simulink model "SimulazioneCaso1_Ins_Sin"  (R2019b)
settings: Solver=VariableStepAuto  StartTime=0.0  StopTime=100  RelTol=1e-3
settings Model: Creator=sugam  LastModifiedBy=sugam

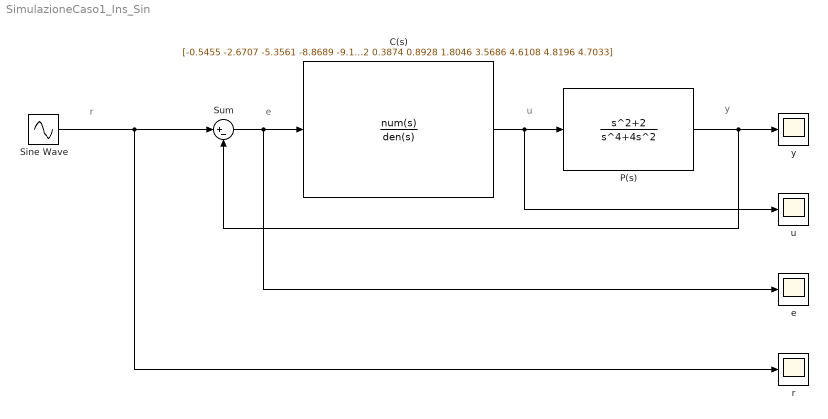
== system SimulazioneCaso1_Ins_Sin ==
  note: y
  note: u
  note: e
  note: r
  C(s) : TransferFcn  Numerator=[-0.5455 -2.6707 -5.3561 -8.8689 -9.1461 0.0529 0.0049]  Denominator=[0.0001 0.0021 0.0197 0.1092 0.3874 0.8928 1.8046 3.5686 4.6108 4.8196 4.7033]
  P(s) : TransferFcn  Numerator=[1 0 2]  Denominator=[1 0 4 0 0]
  Sine Wave : Sin  Amplitude=2  SampleTime=0
  Sum : Sum  Inputs=|+-
  e : Scope
  r : Scope
  u : Scope
  y : Scope
  wires:
  P(s)/1 -> Sum/2, y/1
  Sine Wave/1 -> r/1, Sum/1
  Sum/1 -> e/1, C(s)/1
  C(s)/1 -> u/1, P(s)/1
